simulink model "Reversing_light"  (R2020a)
settings: Solver=FixedStepDiscrete  StartTime=0.0  StopTime=inf  FixedStep=1e-3  MaxStep=1e-3  RelTol=1e-3  EnableMultiTasking=on
libraries: arduinolib x5, dspswit3 x3, simulink x1
settings Model: SILPILModeSetting=veronly  ExtModeTrigDuration=2  Creator=Administrator  LastModifiedBy=Administrator
settings SolverCC: AutoInsertRateTranBlk=on
settings OptimizationCC: DefaultParameterBehavior=Inlined  UseDivisionForNetSlopeComputation=on  GainParamInheritBuiltInType=on  UseFloatMulNetSlope=on  InlineInvariantSignals=on  PassReuseOutputArgsAs=Individual arguments  ZeroExternalMemoryAtStartup=off  ZeroInternalMemoryAtStartup=off  NoFixptDivByZeroProtection=on  EfficientFloat2IntCast=on  LifeSpan=1  MaxStackSize=64  OptimizeBlockOrder=speed  DifferentSizesBufferReuse=on  EfficientTunableParamExpr=on
settings DebuggingCC: MultiTaskRateTransMsg=warning  ParameterTunabilityLossMsg=error
settings HardwareCC: ProdBitPerInt=16  ProdBitPerPointer=16  ProdBitPerSizeT=16  ProdBitPerPtrDiffT=16  ProdLargestAtomicFloat=None  ProdWordSize=8  ProdLongLongMode=on  ProdHWDeviceType=Atmel->AVR
settings SFSimCC: MATLABDynamicMemAlloc=off
settings RTWCC: SystemTargetFile=ert.tlc  HardwareBoard=Arduino Uno  TLCOptions=-aInlineSetEventsForThisBaseRateFcn=TLC_FALSE -aSuppressMultiTaskScheduler=TLC_FALSE -aRateBasedStepFcn=1  TemplateMakefile=ert_default_tmf  Toolchain=Arduino AVR  BuildConfiguration=Faster Runs
settings CodeAppCC: ForceParamTrailComments=on  IgnoreCustomStorageClasses=off  OperatorAnnotations=on  SimulinkDataObjDesc=on  SFDataObjDesc=on  CustomSymbolStrGlobalVar=rt$N$M  CustomSymbolStrType=$N$M  CustomSymbolStrFcn=$N$M$F  CustomSymbolStrMacro=$N$M  InsertBlockDesc=on
settings ERTTargetCC: IncludeMdlTerminateFcn=off  CombineSignalStateStructs=on  SupportAbsoluteTime=off  SupportComplex=off  SupportNonInlinedSFcns=on  ExtModeStaticAllocSize=250  InlinedParameterPlacement=NonHierarchical  ERTFilePackagingFormat=CompactWithDataFile

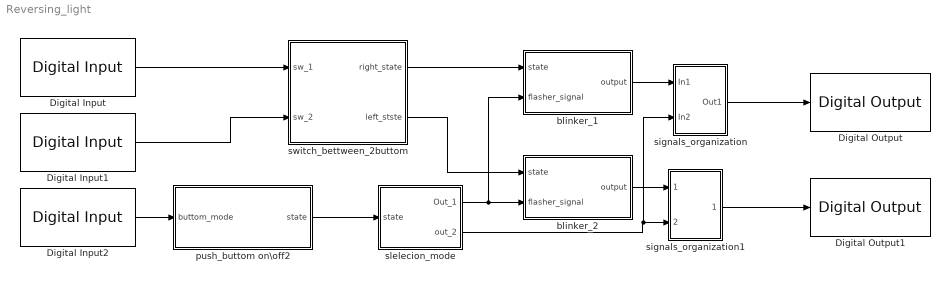
== system Reversing_light ==
  Digital Input : arduinolib/Digital Input  pinNumber=2  Direction=input  SampleTime=.01  blockPlatform=arduino
  Digital Input1 : arduinolib/Digital Input  pinNumber=3  Direction=input  SampleTime=.01  blockPlatform=arduino
  Digital Input2 : arduinolib/Digital Input  pinNumber=4  Direction=input  SampleTime=.01  blockPlatform=arduino
  Digital Output : arduinolib/Digital Output  pinNumber=9  Direction=output  blockPlatform=arduino
  Digital Output1 : arduinolib/Digital Output  pinNumber=10  Direction=output  blockPlatform=arduino
  blinker_1 : Subsystem
  blinker_2 : Subsystem
  push_buttom on\off2 : Subsystem
  signals_organization : Subsystem
  signals_organization1 : Subsystem
  slelecion_mode : Subsystem
  switch_bettween_2buttom : Subsystem
  wires:
  switch_bettween_2buttom/2(left_stste) -> blinker_2/1(state)
  switch_bettween_2buttom/1(right_state) -> blinker_1/1(state)
  Digital Input1/1 -> switch_bettween_2buttom/2(sw_2)
  signals_organization1/1(Out1) -> Digital Output1/1
  blinker_2/1(output) -> signals_organization1/1(output)
  signals_organization/1(Out1) -> Digital Output/1
  Digital Input/1 -> switch_bettween_2buttom/1(sw_1)
  blinker_1/1(output) -> signals_organization/1(In1)
  slelecion_mode/2(out_2) -> signals_organization/2(In2), signals_organization1/2(out_2)
  push_buttom on\off2/1(state) -> slelecion_mode/1(state)
  Digital Input2/1 -> push_buttom on\off2/1(buttom_mode)
  slelecion_mode/1(Out_1) -> blinker_1/2(flasher_signal), blinker_2/2(flasher_signal)

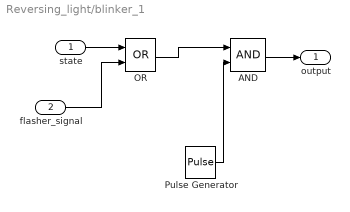
== system Reversing_light/blinker_1 ==
  state : Inport
  flasher_signal : Inport  Port=2
  AND : Logic  AllPortsSameDT=off  OutDataTypeStr=boolean
  OR : Logic  Operator=OR  AllPortsSameDT=off  OutDataTypeStr=boolean
  Pulse Generator : DiscretePulseGenerator  PulseType=Time based  Period=.25  PulseWidth=50
  output : Outport
  wires:
  Pulse Generator/1 -> AND/2
  AND/1 -> output/1
  state/1 -> OR/1
  OR/1 -> AND/1
  flasher_signal/1 -> OR/2

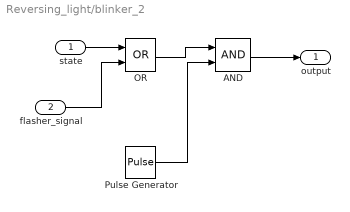
== system Reversing_light/blinker_2 ==
  state : Inport
  flasher_signal : Inport  Port=2
  AND : Logic  AllPortsSameDT=off  OutDataTypeStr=boolean
  OR : Logic  Operator=OR  AllPortsSameDT=off  OutDataTypeStr=boolean
  Pulse Generator : DiscretePulseGenerator  PulseType=Time based  Period=.25  PulseWidth=50
  output : Outport
  wires:
  flasher_signal/1 -> OR/2
  OR/1 -> AND/1
  state/1 -> OR/1
  AND/1 -> output/1
  Pulse Generator/1 -> AND/2

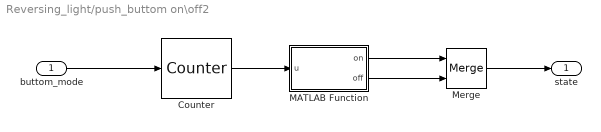
== system Reversing_light/push_buttom on\off2 ==
  buttom_mode : Inport
  Counter : dspswit3/Counter  Direction=Up  CountEvent=Rising edge  CounterSize=User defined  MaxCount=255  InitialCount=1  Output=Count  HitValue=32  ResetInput=off  SamplesPerFrame=1  Ts=1  CntDtype=double  HitDtype=Logical
  MATLAB Function : MATLAB Function  TreatAsAtomicUnit=on
  Merge : Merge
  state : Outport
  wires:
  Counter/1 -> MATLAB Function/1(u)
  MATLAB Function/2(off) -> Merge/2
  MATLAB Function/1(on) -> Merge/1
  Merge/1 -> state/1
  buttom_mode/1 -> Counter/1

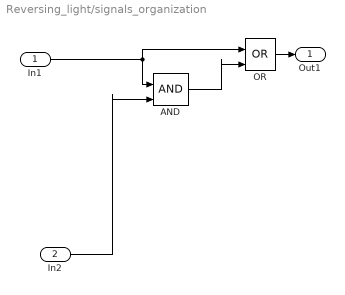
== system Reversing_light/signals_organization ==
  In1 : Inport
  In2 : Inport  Port=2
  AND : Logic  IconShape=distinctive  AllPortsSameDT=off  OutDataTypeStr=boolean
  OR : Logic  Operator=OR  IconShape=distinctive  AllPortsSameDT=off  OutDataTypeStr=boolean
  Out1 : Outport
  wires:
  In1/1 -> OR/1, AND/1
  OR/1 -> Out1/1
  AND/1 -> OR/2
  In2/1 -> AND/2

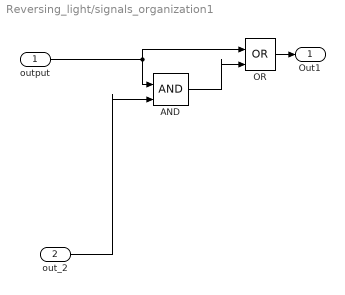
== system Reversing_light/signals_organization1 ==
  output : Inport
  out_2 : Inport  Port=2
  AND : Logic  IconShape=distinctive  AllPortsSameDT=off  OutDataTypeStr=boolean
  OR : Logic  Operator=OR  IconShape=distinctive  AllPortsSameDT=off  OutDataTypeStr=boolean
  Out1 : Outport
  wires:
  out_2/1 -> AND/2
  AND/1 -> OR/2
  OR/1 -> Out1/1
  output/1 -> AND/1, OR/1

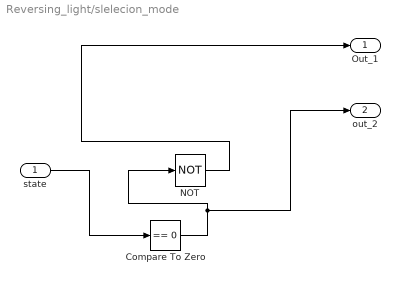
== system Reversing_light/slelecion_mode ==
  state : Inport
  Compare To Zero : simulink/Logic and Bit Operations/Compare To Zero  relop===  OutDataTypeStr=boolean
  NOT : Logic  Operator=NOT  IconShape=distinctive  AllPortsSameDT=off  OutDataTypeStr=boolean
  Out_1 : Outport
  out_2 : Outport  Port=2
  wires:
  Compare To Zero/1 -> out_2/1, NOT/1
  state/1 -> Compare To Zero/1
  NOT/1 -> Out_1/1

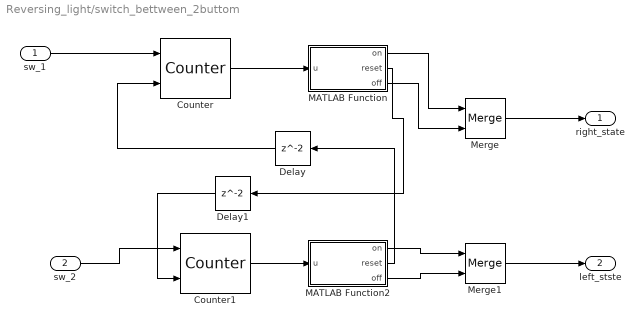
== system Reversing_light/switch_bettween_2buttom ==
  sw_1 : Inport
  sw_2 : Inport  Port=2
  Counter : dspswit3/Counter  Direction=Up  CountEvent=Rising edge  CounterSize=User defined  MaxCount=255  InitialCount=1  Output=Count  HitValue=32  ResetInput=on  SamplesPerFrame=1  Ts=1  CntDtype=double  HitDtype=Logical
  Counter1 : dspswit3/Counter  Direction=Up  CountEvent=Rising edge  CounterSize=User defined  MaxCount=255  InitialCount=1  Output=Count  HitValue=32  ResetInput=on  SamplesPerFrame=1  Ts=1  CntDtype=double  HitDtype=Logical
  Delay : Delay
  Delay1 : Delay
  MATLAB Function : MATLAB Function  TreatAsAtomicUnit=on
  MATLAB Function2 : MATLAB Function  TreatAsAtomicUnit=on
  Merge : Merge
  Merge1 : Merge
  right_state : Outport
  left_stste : Outport  Port=2
  wires:
  Merge1/1 -> left_stste/1
  Delay1/1 -> Counter1/2
  MATLAB Function/2(reset) -> Delay1/1
  Counter/1 -> MATLAB Function/1(u)
  MATLAB Function/3(off) -> Merge/2
  sw_2/1 -> Counter1/1
  Counter1/1 -> MATLAB Function2/1(u)
  MATLAB Function/1(on) -> Merge/1
  MATLAB Function2/3(off) -> Merge1/2
  MATLAB Function2/2(reset) -> Delay/1
  sw_1/1 -> Counter/1
  Delay/1 -> Counter/2
  MATLAB Function2/1(on) -> Merge1/1
  Merge/1 -> right_state/1

== matlab function Reversing_light/push_buttom on\off2/MATLAB Function ==
  data: u input; on output; off output
function [on, off] = fcn(u)
if rem(u,2) ==0
    on=0;
    off=1;
else
    on=1;
    off=0;
end
y = u;

== matlab function Reversing_light/switch_bettween_2buttom/MATLAB Function2 ==
  data: u input; on output; reset output; off output
function [on,reset,off] = fcn(u)
if rem(u,2) ==0
    on=0;
    reset=1;
    off=1;
else
    on=1;
    reset=0;
    off=0;
end
y = u;

== matlab function Reversing_light/switch_bettween_2buttom/MATLAB Function ==
  data: u input; on output; reset output; off output
function [on,reset,off] = fcn(u)
if rem(u,2) ==0
    on=0;
    reset=1;
    off=1;
else
    on=1;
    reset=0;
    off=0;
end
y = u;
